simulink model "M4_Control"  (R2026a)
settings: Solver=FixedStepDiscrete  FixedStep=0.1
PreLoadFcn:
  | createM4BusObjects
values from neighbouring files (symbols this model uses):
  m4StubCmd = Simulink.Bus.createMATLABStruct('SihControlCmdBus')    [createM4BusObjects.m]
settings Model: Creator=jeevan  LastModifiedBy=jeevan

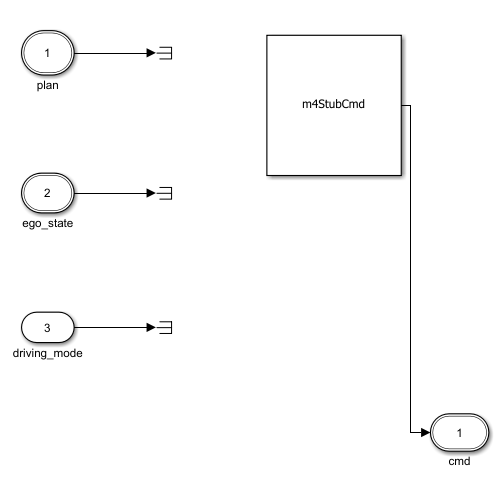
[thumbnail: Simulink's stored preview of the top-level diagram]
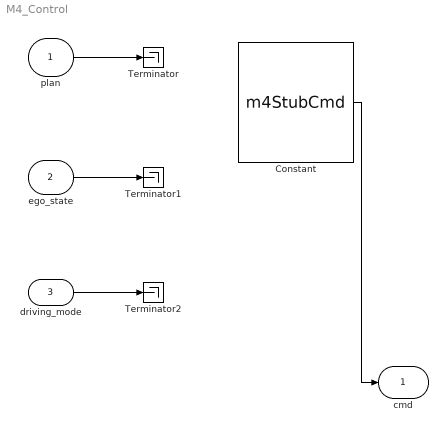
== system M4_Control ==
  plan : Inport  OutDataTypeStr=Bus: SihPlanBus  BusOutputAsStruct=on
  ego_state : Inport  Port=2  OutDataTypeStr=Bus: SihEgoStateBus  BusOutputAsStruct=on
  driving_mode : Inport  Port=3  OutDataTypeStr=Enum: DrivingMode  BusOutputAsStruct=on
  Constant : Constant  Value=m4StubCmd  OutDataTypeStr=Bus: SihControlCmdBus
  Terminator : Terminator
  Terminator1 : Terminator
  Terminator2 : Terminator
  cmd : Outport  OutDataTypeStr=Bus: SihControlCmdBus  BusOutputAsStruct=on
  wires:
  Constant/1 -> cmd/1
  plan/1 -> Terminator/1
  ego_state/1 -> Terminator1/1
  driving_mode/1 -> Terminator2/1
